simulink model "ysw3_43"  (R2014a)
settings: Solver=ode45  StartTime=0.0  StopTime=10.0  RelTol=1e-3
settings Model: Creator=Administrator  LastModifiedBy=Administrator

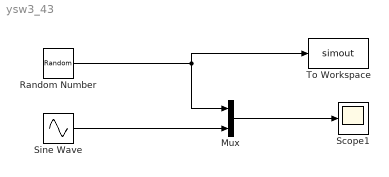
== system ysw3_43 ==
  Mux : Mux  Inputs=2
  Random Number : RandomNumber  Mean=-2  SampleTime=0.1
  Scope1 : Scope
      settings: TimeRange=10
  Sine Wave : Sin  SampleTime=0.1
  To Workspace : ToWorkspace  VariableName=simout  SaveFormat=Timeseries  SampleTime=-1
  wires:
  Random Number/1 -> Mux/1, To Workspace/1
  Sine Wave/1 -> Mux/2
  Mux/1 -> Scope1/1
